simulink model "pulse_model_simulink"  (R2021a)
settings: Solver=VariableStepAuto  StartTime=0.0  StopTime=10.0  RelTol=1e-3
settings Model: Creator=honeycomb0  LastModifiedBy=honeycomb0

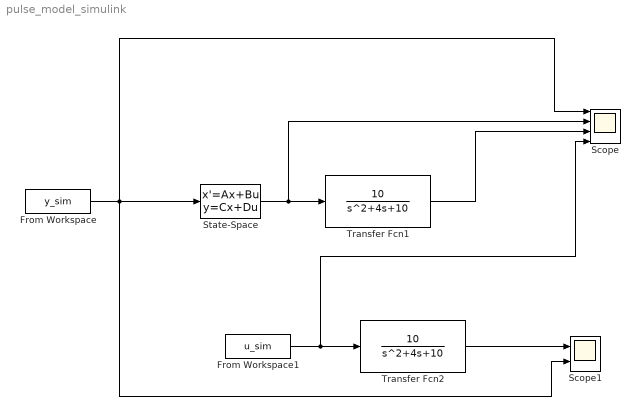
== system pulse_model_simulink ==
  From Workspace : FromWorkspace  VariableName=y_sim  OutputAfterFinalValue=Setting to zero
  From Workspace1 : FromWorkspace  VariableName=u_sim  OutputAfterFinalValue=Setting to zero
  Scope : Scope  NumInputPorts=4
  Scope1 : Scope  NumInputPorts=2
  State-Space : StateSpace  A=|  B=|  C="[2.20179844565148\t0.214096032609243\t-0.400769444435705\t-0.0618393555494560]"  D=0  InitialCondition=|
      A=|
      | [-8.3700   16.4558   10.5765  -10.1209;
      |    46.0697 -160.0626  -95.4121   46.9158;
      |    10.2222   -4.4545  -15.1259   -8.9542;
      |    -9.8918   57.9195   58.9931  -18.1377]
      B=|
      | [-218.884250134802;
      | 2203.82892033210;
      | 48.9264017403017;
      | -685.108241250789]
      InitialCondition=|
      | [-0.1032
      |     2.6374
      |    -2.6731
      |    -0.3092]
  Transfer Fcn1 : TransferFcn  Numerator=[10]  Denominator=[1 4 10]
  Transfer Fcn2 : TransferFcn  Numerator=[10]  Denominator=[1 4 10]
  wires:
  Transfer Fcn1/1 -> Scope/3
  From Workspace1/1 -> Scope/4, Transfer Fcn2/1
  Transfer Fcn2/1 -> Scope1/1
  From Workspace/1 -> State-Space/1, Scope1/2, Scope/1
  State-Space/1 -> Scope/2, Transfer Fcn1/1
